simulink model "MRACmodel"  (R2022b)
settings: Solver=VariableStepAuto  StartTime=0.0  StopTime=inf  RelTol=1e-3
undefined symbols (not defined in the file or in its folder): a, a_m, b, b_m, c
settings Model: PacingRate=10  Creator=Sayan  LastModifiedBy=laksh

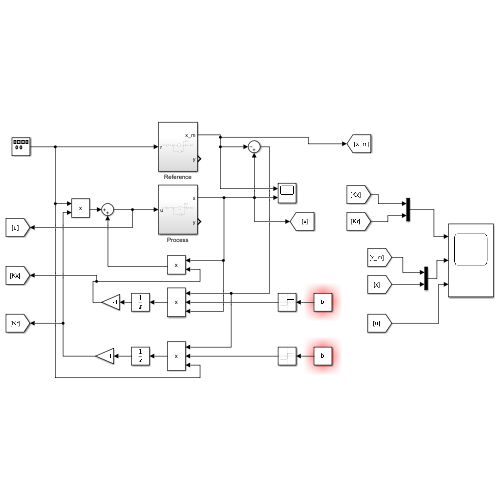
[thumbnail: Simulink's stored preview of the top-level diagram]
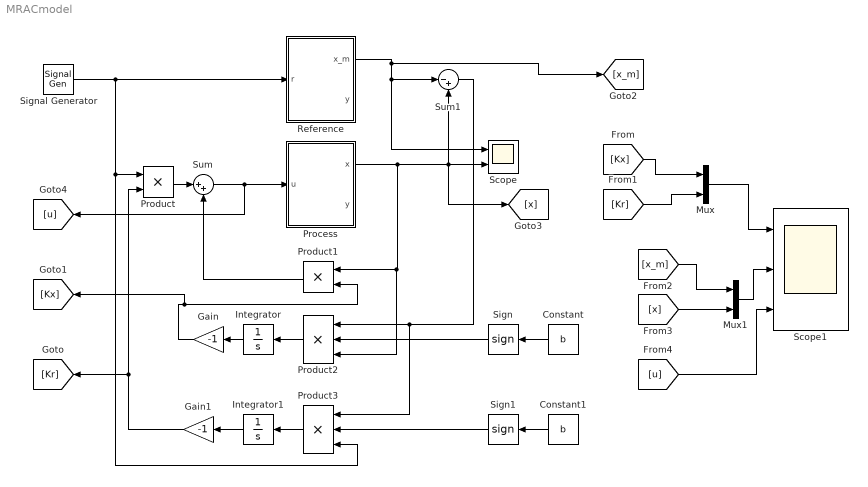
== system MRACmodel ==
  Constant : Constant  Value=b
  Constant1 : Constant  Value=b
  Gain : Gain  Gain=-1
  Gain1 : Gain  Gain=-1
  Integrator : Integrator
  Integrator1 : Integrator
  Mux : Mux  Inputs=2
  Mux1 : Mux  Inputs=2
  Process : Subsystem
  Product : Product
  Product1 : Product
  Product2 : Product  Inputs=3
  Product3 : Product  Inputs=3
  Reference : Subsystem
  Scope : Scope  NumInputPorts=2
  Scope1 : Scope  NumInputPorts=3
  Sign : Signum
  Sign1 : Signum
  Signal Generator : SignalGenerator  WaveForm=square  Frequency=0.2
  Sum : Sum  Inputs=|++
  Sum1 : Sum  Inputs=|-+
  wires:
  Signal Generator/1 -> Reference/1(r), Product3/3, Product/1
  Sum/1 -> [u], Process/1(u)
  Reference/1(x_m) -> [x_m], Scope/1, Sum1/1
  Process/1(x) -> Product2/3, Product1/1, [x], Sum1/2, Scope/2
  Product/1 -> Sum/1
  Product1/1 -> Sum/2
  Sum1/1 -> Product3/1, Product2/1
  Product2/1 -> Integrator/1
  Integrator/1 -> Gain/1
  Gain/1 -> [Kx], Product1/2
  Sign/1 -> Product2/2
  Constant/1 -> Sign/1
  Product3/1 -> Integrator1/1
  Integrator1/1 -> Gain1/1
  Constant1/1 -> Sign1/1
  Sign1/1 -> Product3/2
  Gain1/1 -> [Kr], Product/2
  [Kx] -> Mux/1
  [Kr] -> Mux/2
  Mux/1 -> Scope1/1
  [x_m] -> Mux1/1
  Mux1/1 -> Scope1/2
  [x] -> Mux1/2
  [u] -> Scope1/3

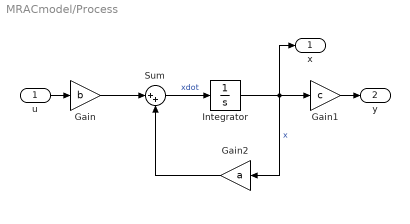
== system MRACmodel/Process ==
  u : Inport
  Gain : Gain  Gain=b
  Gain1 : Gain  Gain=c
  Gain2 : Gain  Gain=a
  Integrator : Integrator
  Sum : Sum  Inputs=|++
  x : Outport
  y : Outport  Port=2
  wires:
  Integrator/1 -> x/1, Gain2/1, Gain1/1  "x"
  Gain2/1 -> Sum/2
  Gain/1 -> Sum/1
  Sum/1 -> Integrator/1  "xdot"
  u/1 -> Gain/1
  Gain1/1 -> y/1

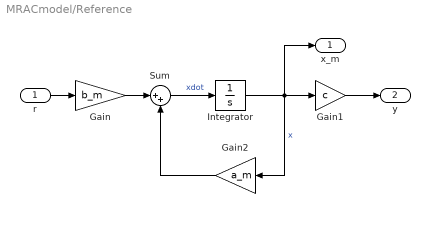
== system MRACmodel/Reference ==
  r : Inport
  Gain : Gain  Gain=b_m
  Gain1 : Gain  Gain=c
  Gain2 : Gain  Gain=a_m
  Integrator : Integrator
  Sum : Sum  Inputs=|++
  x_m : Outport
  y : Outport  Port=2
  wires:
  Integrator/1 -> x_m/1, Gain2/1, Gain1/1  "x"
  r/1 -> Gain/1
  Gain1/1 -> y/1
  Gain2/1 -> Sum/2
  Gain/1 -> Sum/1
  Sum/1 -> Integrator/1  "xdot"
